simulink model "simple_arda"  (R2021b)
settings: Solver=FixedStepAuto  StartTime=0  StopTime=600  RelTol=1e-3
PreLoadFcn:
  | % Setup model parameters
  |                 % Sample time
  |                 %Ts = 0.1;
  |                 % Simulation stop time ("TimeOut")
  |                 %stop_time = 8000;
  |                 % Temperature
  |                 %T_init = 20 + 273.1755;
  |                % T_final = 294.1755;
  |               %  T_env = 20 + 273.15; %#ok<*NASGU>
  |              %   % Heater
  |                 %u_volts_heater_init = 0; % volts
  |                 % Pressure
  |                 %p_init = 101.325; % kPa
  |                 %p_env = 101.325; % kPa
  |                 % Relative humidity and steam
  |                 %phi_init = 0.4987;
  |                 %phi_final = 0.6;
  |                 %phi_env = 0.1;
  |                 %u_steam_init = 0;
  |                 %T_steam = 130 + 273.15;
  |                 % Volumetric flow rate
  |                 %u_volts_fan_init = 1;
  |                 %flow_init = 5.8e-3;
  |                 %flow_final = 0.18;
  |                 % Smooth ramp input parameters
  |                 %smooth_step_heater = make_smooth_step(0, T_init, T_final, Ts, stop_time, 'T_g');
  |                 %smooth_step_steam = make_smooth_step(0, phi_init, phi_final, Ts, stop_time, 'phi');
  |                 %smooth_step_fan = make_smooth_step(0, flow_init, flow_final, Ts, stop_time, 'flow');
  |                 % Parameters to vary for linearization
  |                 % Pipes
  |                 %pipe_length1 = 1; % meters
  |                 %pipe_length2 = 1;
  |                 %pipe_length3 = 1;
  |                 %pipe_cross_sectional_area1 = pi*(2*2.54/2)^2; % cm^2
  |                 %pipe_cross_sectional_area2 = pi*(2*2.54/2)^2;
  |                 %pipe_cross_sectional_area3 = pi*(2*2.54/2)^2;
  |                 %pipe_hydraulic_diameter1 = 2*2.54; %cm
  |                 %pipe_hydraulic_diameter2 = 2*2.54; %cm
  |                 %pipe_hydraulic_diameter3 = 2*2.54; %cm
  |                 % Thermal masses
  |                 %thermal_mass1 = 1; % kg
  |                 %thermal_mass2 = 1; % kg
  |                 %thermal_mass3 = 1; % kg
  |                 %thermal_mass4 = 1; % kg
  |                 %thermal_mass5 = 1; % kg
  |                 %specific_heat1 = 447; % J/(K*kg)
  |                 %specific_heat2 = 447; % J/(K*kg)
  |                 %specific_heat3 = 447; % J/(K*kg)
  |                 %specific_heat4 = 447; % J/(K*kg)
  |                 %specific_heat5 = 447; % J/(K*kg)
libraries: simulink x3
settings Model: DataDictionary=data_dictionary1.sldd  Creator=dmeissner  LastModifiedBy=dmeissner
settings SolverCC: ZeroCrossAlgorithm=Adaptive
settings DataIOCC: DSMLogging=off
settings DebuggingCC: ModelReferenceIOMsg=warning  ModelReferenceVersionMismatchMessage=warning  ModelReferenceIOMismatchMessage=warning  ModelReferenceNoExplicitFinalValueMsg=warning

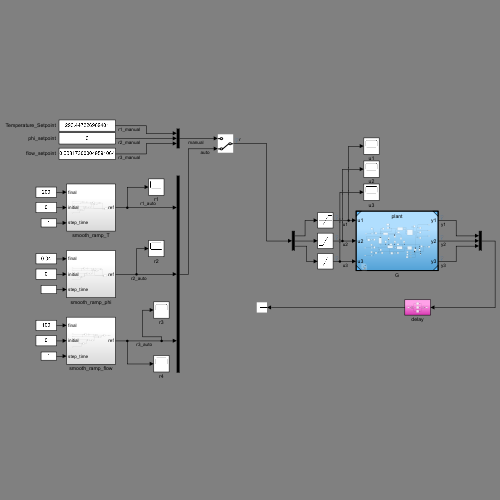
[thumbnail: Simulink's stored preview of the top-level diagram]
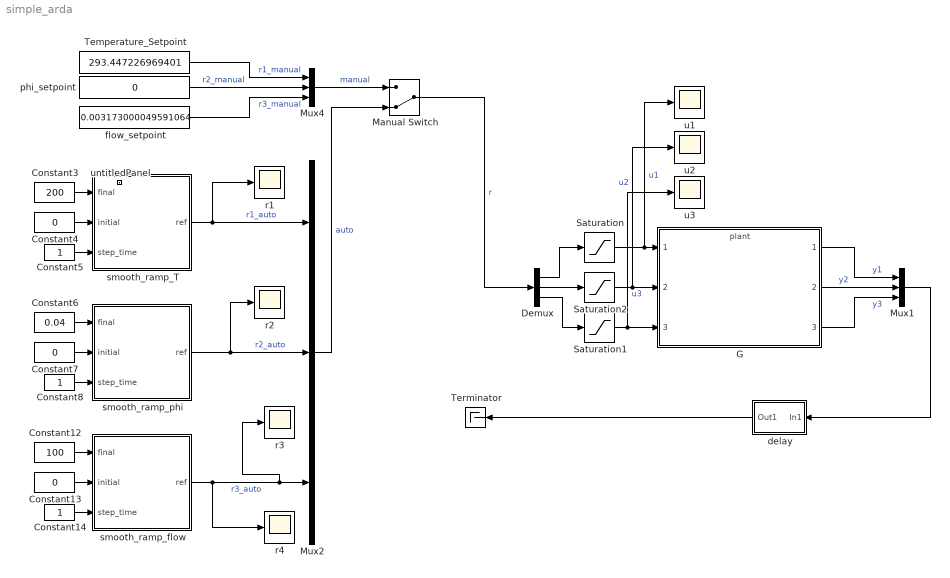
== system simple_arda ==
  Constant12 : Constant  Value=100
  Constant13 : Constant  Value=0
  Constant14 : Constant
  Constant3 : Constant  Value=200
  Constant4 : Constant  Value=0
  Constant5 : Constant
  Constant6 : Constant  Value=0.04
  Constant7 : Constant  Value=0
  Constant8 : Constant
  Demux : Demux  Outputs=3
  G : ModelReference  ModelNameDialog=plant.slx  SimulationMode=Normal  ModelReferenceVersion=1.113
  Manual Switch : ManualSwitch  CurrentSetting=0
  Mux1 : Mux  Inputs=3
  Mux2 : Mux  Inputs=3
  Mux4 : Mux  Inputs=3
  Saturation : Saturate  UpperLimit=460  LowerLimit=0
  Saturation1 : Saturate  UpperLimit=460  LowerLimit=0
  Saturation2 : Saturate  UpperLimit=0.06  LowerLimit=0
  Temperature_Setpoint : Constant  Value=293.447226969401
  Terminator : Terminator
  delay : Subsystem
  flow_setpoint : Constant  Value=0.003173000049591064
  phi_setpoint : Constant  Value=0
  r{1..4} (4 alike) : Scope
  smooth_ramp_T : Subsystem
  smooth_ramp_flow : Subsystem
  smooth_ramp_phi : Subsystem
  u1 : Scope
  u2 : Scope
  u3 : Scope
  untitledPanel : Subsystem  Tag=HiddenForWebPanel  IsWebBlockPanel=on
  wires:
  Temperature_Setpoint/1 -> Mux4/1  "r1_manual"
  G/2 -> Mux1/2  "y2"
  G/1 -> Mux1/1  "y1"
  G/3 -> Mux1/3  "y3"
  Saturation/1 -> u1/1, G/1  "u1"
  Saturation2/1 -> u2/1, G/2  "u2"
  Saturation1/1 -> u3/1, G/3  "u3"
  Mux1/1 -> delay/1(In1)
  delay/1(Out1) -> Terminator/1
  phi_setpoint/1 -> Mux4/2  "r2_manual"
  flow_setpoint/1 -> Mux4/3  "r3_manual"
  Mux4/1 -> Manual Switch/1  "manual"
  Manual Switch/1 -> Demux/1  "r"
  smooth_ramp_phi/1(ref) -> Mux2/2, r2/1  "r2_auto"
  smooth_ramp_T/1(ref) -> r1/1, Mux2/1  "r1_auto"
  smooth_ramp_flow/1(ref) -> r4/1, r3/1, Mux2/3  "r3_auto"
  Mux2/1 -> Manual Switch/2  "auto"
  Constant5/1 -> smooth_ramp_T/3(step_time)
  Constant4/1 -> smooth_ramp_T/2(initial)
  Constant3/1 -> smooth_ramp_T/1(final)
  Constant6/1 -> smooth_ramp_phi/1(final)
  Constant8/1 -> smooth_ramp_phi/3(step_time)
  Constant7/1 -> smooth_ramp_phi/2(initial)
  Constant13/1 -> smooth_ramp_flow/2(initial)
  Constant14/1 -> smooth_ramp_flow/3(step_time)
  Constant12/1 -> smooth_ramp_flow/1(final)
  Demux/1 -> Saturation/1
  Demux/2 -> Saturation2/1
  Demux/3 -> Saturation1/1

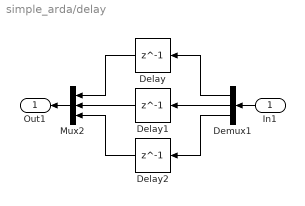
== system simple_arda/delay ==
  In1 : Inport
  Delay : Delay  DelayLength=1
  Delay1 : Delay  DelayLength=1
  Delay2 : Delay  DelayLength=1
  Demux1 : Demux  Outputs=3
  Mux2 : Mux  Inputs=3
  Out1 : Outport
  wires:
  Mux2/1 -> Out1/1
  Demux1/2 -> Delay1/1
  In1/1 -> Demux1/1
  Delay1/1 -> Mux2/2
  Demux1/3 -> Delay2/1
  Delay/1 -> Mux2/1
  Demux1/1 -> Delay/1
  Delay2/1 -> Mux2/3

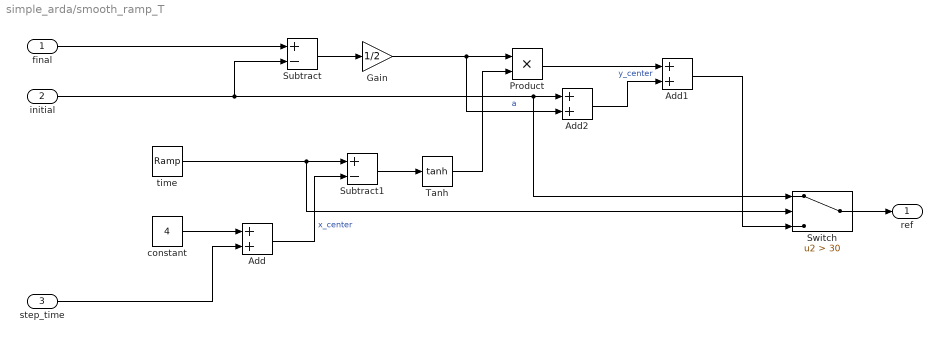
== system simple_arda/smooth_ramp_T ==
  final : Inport
  initial : Inport  Port=2
  step_time : Inport  Port=3
  Add : Sum
  Add1 : Sum
  Add2 : Sum
  Gain : Gain  Gain=1/2
  Product : Product
  Subtract : Sum  Inputs=+-
  Subtract1 : Sum  Inputs=+-
  Switch : Switch  Criteria=u2 > Threshold  Threshold=30
  Tanh : Trigonometry  Operator=tanh
  constant : Constant  Value=4
  time : simulink/Sources/Ramp  slope=1  start=0  InitialOutput=0
  ref : Outport
  wires:
  final/1 -> Subtract/1
  initial/1 -> Switch/1, Add2/1, Subtract/2
  Subtract/1 -> Gain/1
  Gain/1 -> Add2/2, Product/1  "a"
  constant/1 -> Add/1
  step_time/1 -> Add/2
  Add/1 -> Subtract1/2  "x_center"
  time/1 -> Switch/2, Subtract1/1
  Subtract1/1 -> Tanh/1
  Tanh/1 -> Product/2
  Product/1 -> Add1/1
  Add2/1 -> Add1/2  "y_center"
  Switch/1 -> ref/1
  Add1/1 -> Switch/3

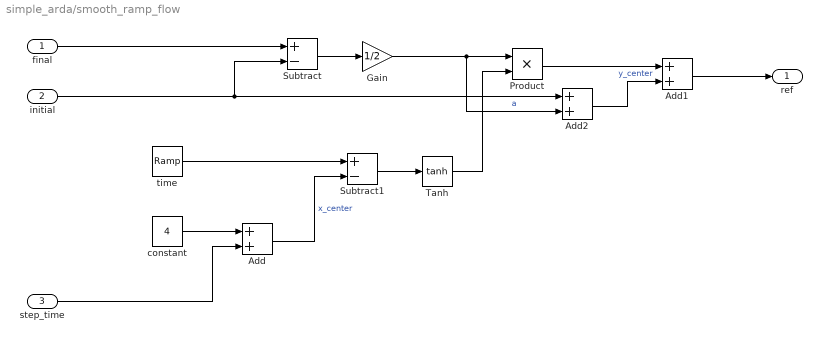
== system simple_arda/smooth_ramp_flow ==
  final : Inport
  initial : Inport  Port=2
  step_time : Inport  Port=3
  Add : Sum
  Add1 : Sum
  Add2 : Sum
  Gain : Gain  Gain=1/2
  Product : Product
  Subtract : Sum  Inputs=+-
  Subtract1 : Sum  Inputs=+-
  Tanh : Trigonometry  Operator=tanh
  constant : Constant  Value=4
  time : simulink/Sources/Ramp  slope=1  start=0  InitialOutput=0
  ref : Outport
  wires:
  final/1 -> Subtract/1
  initial/1 -> Add2/1, Subtract/2
  Subtract/1 -> Gain/1
  Gain/1 -> Add2/2, Product/1  "a"
  constant/1 -> Add/1
  step_time/1 -> Add/2
  Add/1 -> Subtract1/2  "x_center"
  time/1 -> Subtract1/1
  Subtract1/1 -> Tanh/1
  Tanh/1 -> Product/2
  Product/1 -> Add1/1
  Add2/1 -> Add1/2  "y_center"
  Add1/1 -> ref/1

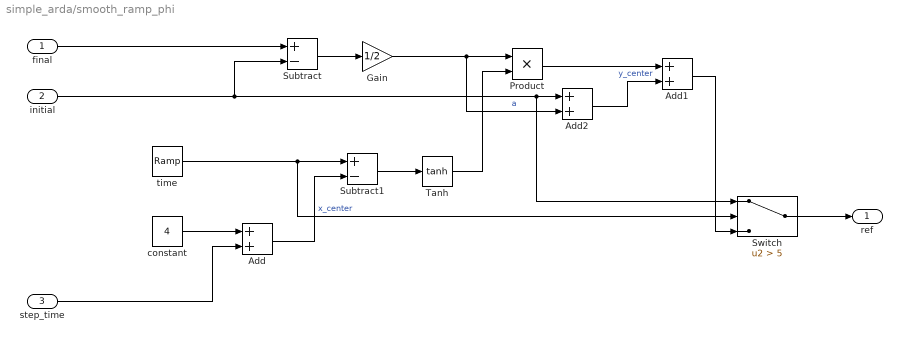
== system simple_arda/smooth_ramp_phi ==
  final : Inport
  initial : Inport  Port=2
  step_time : Inport  Port=3
  Add : Sum
  Add1 : Sum
  Add2 : Sum
  Gain : Gain  Gain=1/2
  Product : Product
  Subtract : Sum  Inputs=+-
  Subtract1 : Sum  Inputs=+-
  Switch : Switch  Criteria=u2 > Threshold  Threshold=5
  Tanh : Trigonometry  Operator=tanh
  constant : Constant  Value=4
  time : simulink/Sources/Ramp  slope=1  start=0  InitialOutput=0
  ref : Outport
  wires:
  final/1 -> Subtract/1
  initial/1 -> Switch/1, Add2/1, Subtract/2
  Subtract/1 -> Gain/1
  Gain/1 -> Add2/2, Product/1  "a"
  constant/1 -> Add/1
  step_time/1 -> Add/2
  Add/1 -> Subtract1/2  "x_center"
  time/1 -> Switch/2, Subtract1/1
  Subtract1/1 -> Tanh/1
  Tanh/1 -> Product/2
  Product/1 -> Add1/1
  Add2/1 -> Add1/2  "y_center"
  Switch/1 -> ref/1
  Add1/1 -> Switch/3

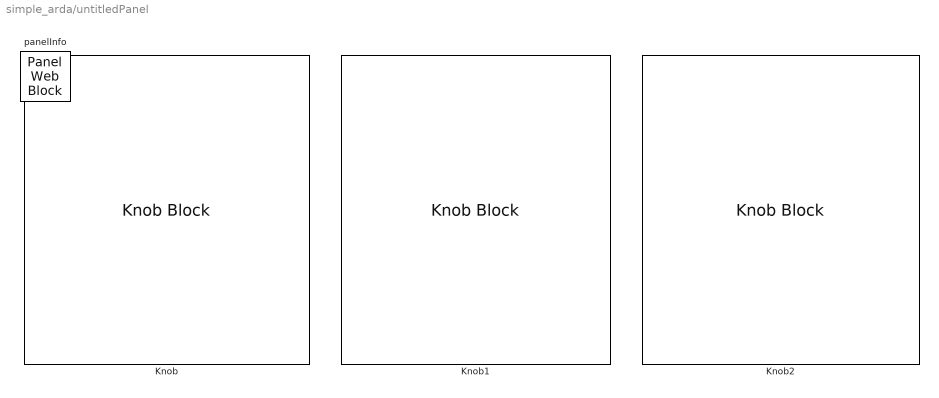
== system simple_arda/untitledPanel ==
  Knob : KnobBlock  Tag=HiddenForWebPanel  PanelInfo="{\"panelId\":\"panelId-06cae6c1-80a6-464e-a568-f56bf80fba14\",\"type\":\"panelChild\",\"version\":\"2019b\",\"zIndex\":1500004}"  ScaleMin=290  ScaleMax=450  TickInterval=10
  Knob1 : KnobBlock  Tag=HiddenForWebPanel  PanelInfo="{\"panelId\":\"panelId-06cae6c1-80a6-464e-a568-f56bf80fba14\",\"type\":\"panelChild\",\"version\":\"2019b\",\"zIndex\":1500002}"  ScaleMax=1  TickInterval=0.1
  Knob2 : KnobBlock  Tag=HiddenForWebPanel  PanelInfo="{\"panelId\":\"panelId-06cae6c1-80a6-464e-a568-f56bf80fba14\",\"type\":\"panelChild\",\"version\":\"2019b\",\"zIndex\":1500006}"  ScaleMax=0.18  TickInterval=0.01
  panelInfo : PanelWebBlock  Tag=HiddenForWebPanel  PanelInfo="{\"compacted\":true,\"height\":349,\"isActiveTab\":true,\"left\":40,\"name\":\"Panel\",\"panelId\":\"panelId-06cae6c1-80a6-464e-a568-f56bf80fba14\",\"tabIndex\":0,\"tabbedSetId\":\"tabbedSet4008599384\",\"top\":58,\"type\":\"panel\",\"version\":\"2019b\",\"visible\":true,\"width\":935,\"zIndex\":1500002}"  PanelSnapshot=<binary blob, 164088 chars, not shown>
